simulink model "duffing_new"  (R2022a)
settings: Solver=FixedStepAuto  StartTime=0.0  StopTime=8  FixedStep=Ts  RelTol=1e-3
model workspace (MAT data in the model file):
  B = Simulink.Parameter
  B.Value = 1
  B.DataType = 'auto'
  B.Complexity = 'real'
  B.Dimensions = [1 1]
  Sig = Simulink.Signal
  Sig.DataType = 'auto'
  Sig.Dimensions = -1
  Sig.DimensionsMode = 'auto'
  Sig.Complexity = 'auto'
  Sig.SampleTime = -1
  Sig.SamplingMode = 'auto'
  Ts = Simulink.Parameter
  Ts.Value = 0.01
  Ts.DataType = 'auto'
  Ts.Complexity = 'real'
  Ts.Dimensions = [1 1]
  a = Simulink.Parameter
  a.Value = -1
  a.DataType = 'auto'
  a.Complexity = 'real'
  a.Dimensions = [1 1]
  d = Simulink.Parameter
  d.Value = 0.3
  d.DataType = 'auto'
  d.Complexity = 'real'
  d.Dimensions = [1 1]
  lamda = Simulink.Parameter
  lamda.Value = 0.37
  lamda.DataType = 'auto'
  lamda.Complexity = 'real'
  lamda.Dimensions = [1 1]
  w = Simulink.Parameter
  w.Value = 1.2
  w.DataType = 'auto'
  w.Complexity = 'real'
  w.Dimensions = [1 1]
settings Model: Creator=xzhao  LastModifiedBy=xzhao

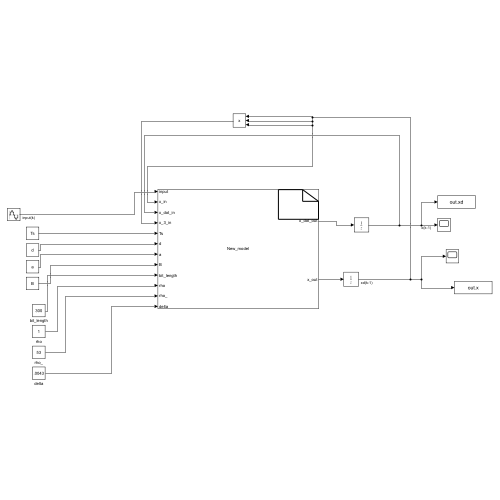
[thumbnail: Simulink's stored preview of the top-level diagram]
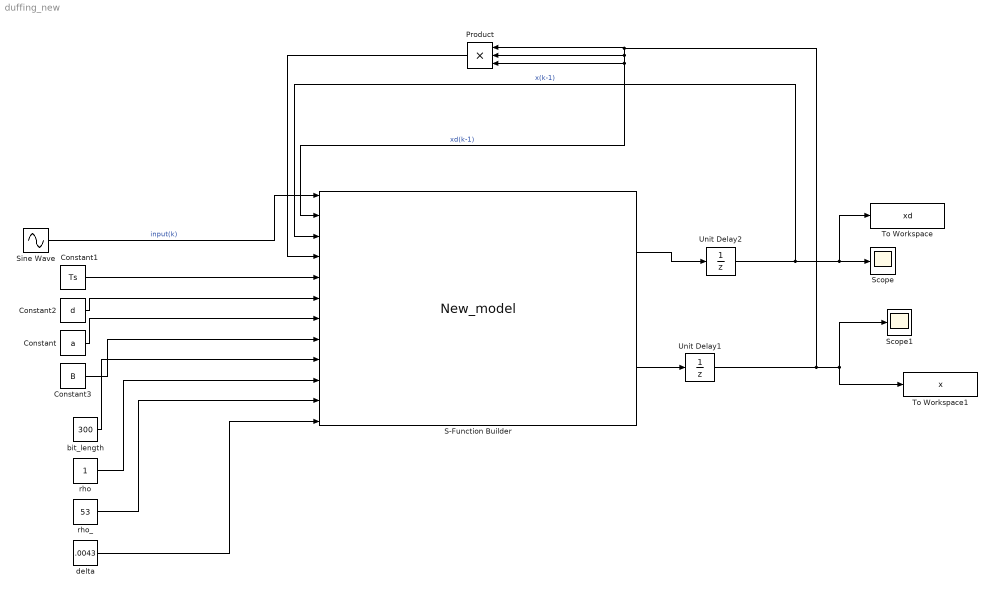
== system duffing_new ==
  Constant : Constant  Value=a
  Constant1 : Constant  Value=Ts
  Constant2 : Constant  Value=d
  Constant3 : Constant  Value=B
  Product : Product  Inputs=3
  S-Function Builder : S-Function  FunctionName=New_model  SFunctionModules=New_model_wrapper  SFunctionDeploymentMode=off  EnableBusSupport=off  mask(S-Function Builder){}
      mask help: Simulink:masks:SFunctionBuilder_MD
      mask init:
      | val = [[.9  0.75 0.75 1 1 .9 .9 1]',[1 1 0.75 0.75 .9 .9 1 .9]'];try , sys = get_param(gcb,'SfunBuilderFcnName');if isempty(sys), sys = get_param(gcb,'FunctionName'); end,catch, sys = get_param(gcb,'FunctionName'); end
      settings: CopyFcn=set_param(gcbh,'LinkStatus','none')  OpenFcn=sfunctionwizard(gcbh)
      mask Display:
      | plot(val(:,1),val(:,2))
      | disp(sys)
      | port_label('input',1,'input')
      | port_label('input',2,'x_in')
      | port_label('input',3,'x_dot_in')
      | port_label('input',4,'x_3_in')
      | port_label('input',5,'Ts')
      | port_label('input',6,'d')
      | port_label('input',7,'a')
      | port_label('input',8,'B')
      | port_label('input',9,'bit_length')
      | port_label('input',10,'rho')
      | port_label('input',11,'rho_')
      | port_label('input',12,'delta')
      | port_label('output',1,'x_dot_out')
      | port_label('output',2,'x_out')
  Scope : Scope
  Scope1 : Scope
  Sine Wave : Sin  Amplitude=lamda  Frequency=w  Phase=w*pi/2  SampleTime=Ts
  To Workspace : ToWorkspace  VariableName=xd  SaveFormat=Timeseries  SampleTime=-1
  To Workspace1 : ToWorkspace  VariableName=x  SaveFormat=Timeseries  SampleTime=-1
  Unit Delay1 : UnitDelay  InitialCondition=1  SampleTime=Ts  HasFrameUpgradeWarning=on
  Unit Delay2 : UnitDelay  SampleTime=-1  HasFrameUpgradeWarning=on
  bit_length : Constant  Value=300
  delta : Constant  Value=.0043
  rho : Constant
  rho_ : Constant  Value=53
  wires:
  Sine Wave/1 -> S-Function Builder/1  "input(k)"
  S-Function Builder/1 -> Unit Delay2/1
  Unit Delay1/1 -> S-Function Builder/2, Product/3, Product/2, Product/1, Scope1/1, To Workspace1/1  "xd(k-1)"
  Product/1 -> S-Function Builder/4
  Unit Delay2/1 -> S-Function Builder/3, To Workspace/1, Scope/1  "x(k-1)"
  Constant2/1 -> S-Function Builder/6
  Constant/1 -> S-Function Builder/7
  Constant3/1 -> S-Function Builder/8
  S-Function Builder/2 -> Unit Delay1/1
  Constant1/1 -> S-Function Builder/5
  bit_length/1 -> S-Function Builder/9
  rho/1 -> S-Function Builder/10
  rho_/1 -> S-Function Builder/11
  delta/1 -> S-Function Builder/12
